simulink model "mass_spring_damper_simulink (3)"  (R2024b)
settings: Solver=VariableStepAuto  StartTime=0.0  StopTime=10.0  RelTol=1e-3
undefined symbols (not defined in the file): b1, b2, k1, k2, M1, M2
settings Model: Creator=Asus  LastModifiedBy=Asus

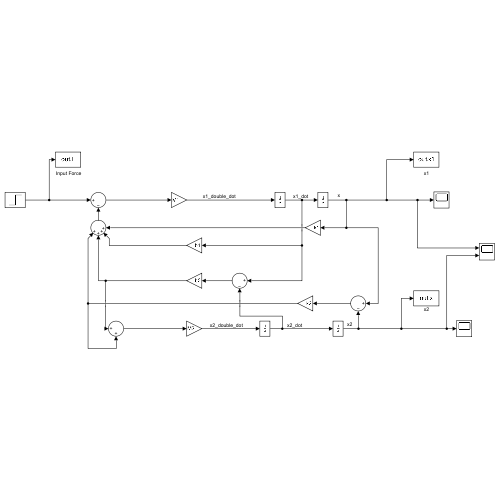
[thumbnail: Simulink's stored preview of the top-level diagram]
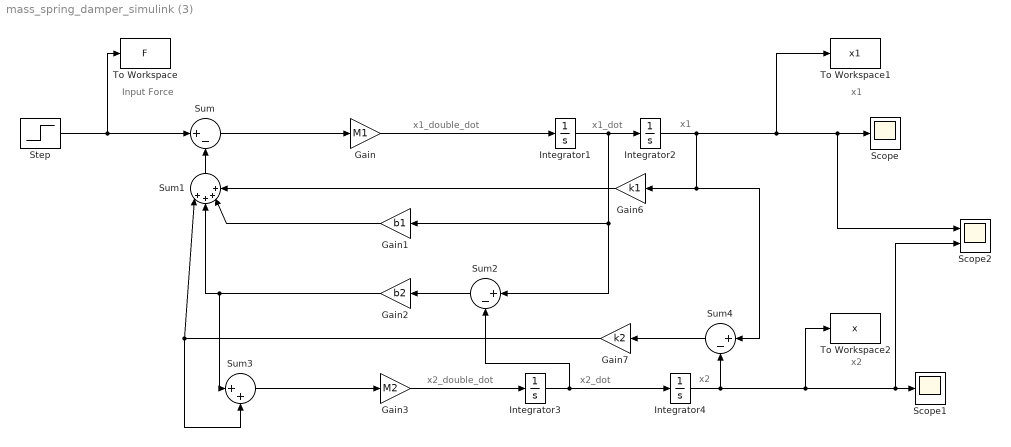
== system mass_spring_damper_simulink (3) ==
  note: x1_dot
  note: x1_double_dot
  note: Input Force
  note: x1
  note: x1
  note: x2
  note: x2_dot
  note: x2_double_dot
  note: x2
  Gain : Gain  Gain=M1
  Gain1 : Gain  Gain=b1
  Gain2 : Gain  Gain=b2
  Gain3 : Gain  Gain=M2
  Gain6 : Gain  Gain=k1
  Gain7 : Gain  Gain=k2
  Integrator{1..4} (4 alike) : Integrator
  Scope : Scope
  Scope1 : Scope
  Scope2 : Scope  NumInputPorts=2
  Step : Step  SampleTime=0
  Sum : Sum  Inputs=|+-
  Sum1 : Sum  Inputs=|++++
  Sum2 : Sum  Inputs=|+-
  Sum3 : Sum  Inputs=|++
  Sum4 : Sum  Inputs=|+-
  To Workspace : ToWorkspace  VariableName=F  SaveFormat=Timeseries  SampleTime=-1
  To Workspace1 : ToWorkspace  VariableName=x1  SaveFormat=Timeseries  SampleTime=-1
  To Workspace2 : ToWorkspace  VariableName=x  SaveFormat=Timeseries  SampleTime=-1
  wires:
  Sum1/1 -> Sum/2
  Sum/1 -> Gain/1
  Step/1 -> To Workspace/1, Sum/1
  Gain6/1 -> Sum1/4
  Gain/1 -> Integrator1/1
  Sum2/1 -> Gain2/1
  Gain1/1 -> Sum1/3
  Gain2/1 -> Sum3/1, Sum1/2
  Integrator1/1 -> Sum2/1, Gain1/1, Integrator2/1
  Sum3/1 -> Gain3/1
  Gain3/1 -> Integrator3/1
  Gain7/1 -> Sum1/1, Sum3/2
  Integrator4/1 -> Sum4/2, Scope2/2, Scope1/1, To Workspace2/1
  Integrator2/1 -> Sum4/1, Gain6/1, Scope2/1, Scope/1, To Workspace1/1
  Sum4/1 -> Gain7/1
  Integrator3/1 -> Integrator4/1, Sum2/2
